simulink model "CA1"  (R2024b)
settings: Solver=VariableStepAuto  StartTime=0.0  StopTime=100  RelTol=1e-3
values from neighbouring files (symbols this model uses):
  am = 5    [Parameter.m]
  Ga = diag([12*ga,10*ga,20*ga,200*ga,200*ga])    [Parameter.m]
  Kaster = Km/Kp    (= -10)    [Parameter.m]
  Kp = b0    (= -0.5)    [Parameter.m]
  Rm = [1 am]    [Parameter.m]
  Rp = [1 a1 a2]    [Parameter.m]
  theta_bar_aster = [Kaster, -g2, -g1 , -f2, -f1]    [Parameter.m]
  Tp = [1 2*zeta*wn wn^2]    [Parameter.m]
  Zp = [1 b1/b0]    [Parameter.m]
settings Model: Creator=xym  LastModifiedBy=xym
settings DataIOCC: InitialState=theta_bar_aster  SaveOutput=off

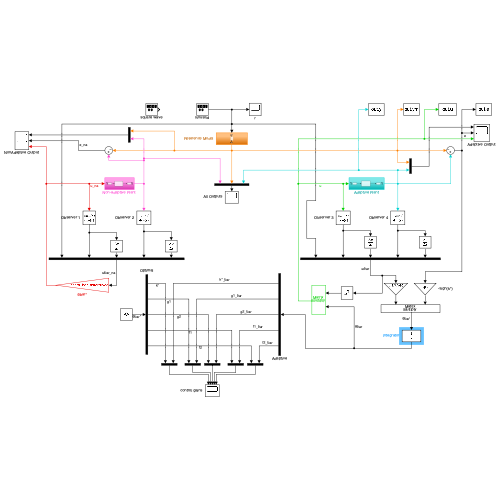
[thumbnail: Simulink's stored preview of the top-level diagram]
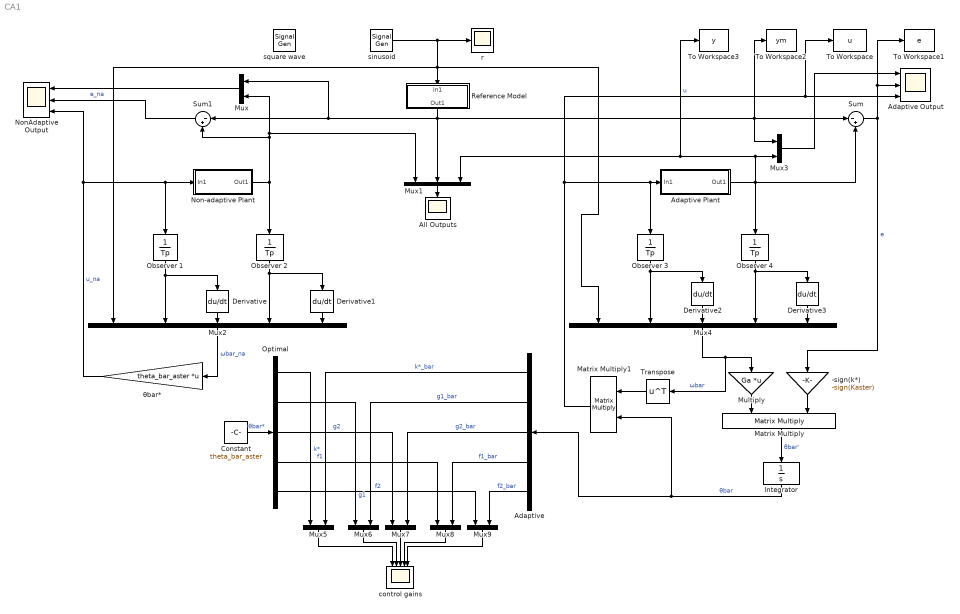
== system CA1 ==
  -sign(k*) : Gain  Gain=-sign(Kaster)
  Adaptive : Demux  Outputs=5
  Adaptive Output : Scope  NumInputPorts=3
  Adaptive Plant : Subsystem
  All Outputs : Scope
  Constant : Constant  Value=theta_bar_aster
  Derivative{,1..3} (4 alike) : Derivative
  Integrator : Integrator  InitialCondition=theta_bar_aster*0.1  ZeroCross=off  ContinuousStateAttributes='theta_bar'
  Matrix Multiply : Product  Multiplication=Matrix(*)
  Matrix Multiply1 : Product  Multiplication=Matrix(*)
  Multiply : Gain  Gain=Ga  Multiplication=Matrix(K*u) (u vector)
  Mux{,3,5..9} (7 alike) : Mux  Inputs=2
  Mux1 : Mux  Inputs=3
  Mux2 : Mux  Inputs=5
  Mux4 : Mux  Inputs=5
  Non-adaptive Plant : Subsystem
  NonAdaptive Output : Scope  NumInputPorts=3
  Observer {1..4} (4 alike) : TransferFcn  Denominator=Tp
  Optimal : Demux  Outputs=5
  Reference Model : Subsystem
  Sum : Sum  Inputs=|-+
  Sum1 : Sum  Inputs=|-+
  To Workspace : ToWorkspace  VariableName=u  SaveFormat=Timeseries  SampleTime=-1
  To Workspace1 : ToWorkspace  VariableName=e  SaveFormat=Timeseries  SampleTime=-1
  To Workspace2 : ToWorkspace  VariableName=ym  SaveFormat=Timeseries  SampleTime=-1
  To Workspace3 : ToWorkspace  VariableName=y  SaveFormat=Timeseries  SampleTime=-1
  Transpose : Math  Operator=transpose
  control gains : Scope  NumInputPorts=5
  r : Scope
  sinusoid : SignalGenerator  Amplitude=10  Frequency=2  Units=rad/sec
  "square wave " : SignalGenerator  WaveForm=square  Frequency=0.1
  θbar* : Gain  Gain=theta_bar_aster  Multiplication=Matrix(K*u) (u vector)
  wires:
  sinusoid/1 -> r/1, Mux4/1, Mux2/1, Reference Model/1(In1)
  Reference Model/1(Out1) -> Mux1/2, Mux/1, Sum1/1, To Workspace2/1, Sum/1, Mux3/1
  Mux1/1 -> All Outputs/1
  Non-adaptive Plant/1(Out1) -> Mux/2, Mux1/1, Sum1/2, Observer 2/1
  Observer 1/1 -> Derivative/1, Mux2/2
  Derivative/1 -> Mux2/3
  Observer 2/1 -> Derivative1/1, Mux2/4
  Derivative1/1 -> Mux2/5
  θbar*/1 -> Non-adaptive Plant/1(In1), Observer 1/1, NonAdaptive Output/3  "u_na"
  Mux3/1 -> Adaptive Output/1
  Observer 3/1 -> Derivative2/1, Mux4/2
  Derivative2/1 -> Mux4/3
  Derivative3/1 -> Mux4/5
  Observer 4/1 -> Derivative3/1, Mux4/4
  Matrix Multiply1/1 -> Adaptive Output/3, To Workspace/1, Adaptive Plant/1(In1), Observer 3/1  "u"
  Adaptive Plant/1(Out1) -> Observer 4/1, To Workspace3/1, Mux1/3, Mux3/2, Sum/2
  Sum/1 -> -sign(k*)/1, Adaptive Output/2, To Workspace1/1  "e"
  Mux4/1 -> Multiply/1, Transpose/1  "ωbar"
  Multiply/1 -> Matrix Multiply/1
  -sign(k*)/1 -> Matrix Multiply/2
  Transpose/1 -> Matrix Multiply1/1
  Matrix Multiply/1 -> Integrator/1  "θbar'"
  Integrator/1 -> Matrix Multiply1/2, Adaptive/1  "θbar"
  Mux2/1 -> θbar*/1  "ωbar_na"
  Constant/1 -> Optimal/1  "θbar*"
  Optimal/1 -> Mux5/1  "k*"
  Adaptive/1 -> Mux5/2  "k*_bar"
  Optimal/2 -> Mux6/1  "g1"
  Adaptive/2 -> Mux6/2  "g1_bar"
  Optimal/3 -> Mux7/1  "g2"
  Optimal/4 -> Mux8/1  "f1"
  Adaptive/4 -> Mux8/2  "f1_bar"
  Optimal/5 -> Mux9/1  "f2"
  Adaptive/5 -> Mux9/2  "f2_bar"
  Mux6/1 -> control gains/2
  Adaptive/3 -> Mux7/2  "g2_bar"
  Mux5/1 -> control gains/1
  Mux7/1 -> control gains/3
  Mux8/1 -> control gains/4
  Mux9/1 -> control gains/5
  Sum1/1 -> NonAdaptive Output/2  "e_na"
  Mux/1 -> NonAdaptive Output/1

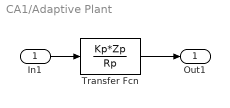
== system CA1/Adaptive Plant ==
  In1 : Inport
  Transfer Fcn : TransferFcn  Numerator=Kp*Zp  Denominator=Rp
  Out1 : Outport
  wires:
  Transfer Fcn/1 -> Out1/1
  In1/1 -> Transfer Fcn/1

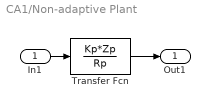
== system CA1/Non-adaptive Plant ==
  In1 : Inport
  Transfer Fcn : TransferFcn  Numerator=Kp*Zp  Denominator=Rp
  Out1 : Outport
  wires:
  Transfer Fcn/1 -> Out1/1
  In1/1 -> Transfer Fcn/1

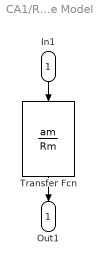
== system CA1/Reference Model ==
  In1 : Inport
  Transfer Fcn : TransferFcn  Numerator=am  Denominator=Rm
  Out1 : Outport
  wires:
  In1/1 -> Transfer Fcn/1
  Transfer Fcn/1 -> Out1/1
